simulink model "Aufgabe2"  (R2018b)
settings: Solver=VariableStepAuto  StartTime=0.0  StopTime=tEnd  RelTol=1e-3
settings Model: Creator=gome  LastModifiedBy=gome

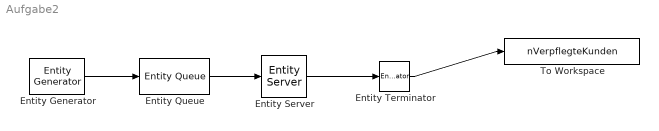
== system Aufgabe2 ==
  Entity Generator : EntityGenerator  OutputPortMessageModes=m  TimeSource=MATLAB action  IntergenerationTimeAction=|  EntityType=Structured  EntityTypeName=Entity
      | persistent z
      | if isempty(z)
      |     z = 0;
      |     rng(1000);
      | end
      | 
      | lambda = 0.3;
      | dt = exprnd(1/lambda);
  Entity Queue : EntityQueue  InputPortMessageModes=m  OutputPortMessageModes=m  Capacity=n
      settings: OutputPortMap=o5
  Entity Server : EntityServer  InputPortMessageModes=m  OutputPortMessageModes=m  Capacity=1  ServiceTimeSource=MATLAB action  ServiceTimeAction=|
      | persistent z
      | if isempty(z)
      |     z = 0;
      |     rng(2000);
      | end
      | 
      | ts = 2;
      | 
      | dt = exprnd(ts);
  Entity Terminator : EntityTerminator  InputPortMessageModes=m  NumberEntitiesArrived=on
      settings: OutputPortMap=o0
  To Workspace : ToWorkspace  VariableName=nVerpflegteKunden  SampleTime=-1
  wires:
  Entity Generator/1 -> Entity Queue/1
  Entity Queue/1 -> Entity Server/1
  Entity Server/1 -> Entity Terminator/1
  Entity Terminator/1 -> To Workspace/1
